simulink model "sensorFusionOfflineHMI"  (R2015b)
settings: Solver=FixedStepDiscrete  StartTime=0.0  StopTime=endTime  FixedStep=0.005  MaxStep=0.005  RelTol=1e-3
values from neighbouring files (symbols this model uses):
  resetStepTime = 500    [main.m]    (also in mainHMI.m)
undefined symbols (not defined in the file or in its folder): EGOSF_CompassHeadingCov, EGOSF_DetectionNorthMax, EGOSF_DetectionNorthMin, EGOSF_GPSHeadingCov, EGOSF_HeadingVelocityLimit, EGOSF_LatAccCov, EGOSF_LatVelInitCov, EGOSF_LonAccCov, EGOSF_LonSpeedCov, EGOSF_OutlierDetection, EGOSF_PhiCov, EGOSF_PhiScale, EGOSF_Pproc, EGOSF_SteeringRatio, EGOSF_YawRateCov, UTMZone
libraries: powerlib_meascontrol x1, sldrtlib x1, etargetslib x1, dspnetwork x1
settings Model: Creator=hultr  LastModifiedBy=axel
settings DataIOCC: SaveFormat=Array
settings DebuggingCC: SolverPrmCheckMsg=warning  InheritedTsInSrcMsg=none  BusObjectLabelMismatch=none
settings HardwareCC: ProdBitPerPointer=32  ProdLargestAtomicFloat=None  ProdIntDivRoundTo=Undefined  ProdEndianess=Unspecified  ProdWordSize=32  ProdHWDeviceType=32-bit Generic
settings GRTTargetCC: GeneratePreprocessorConditionals=Disable all
settings ConfigComp: CovModelRefEnable=Off  CovSFcnEnable=off

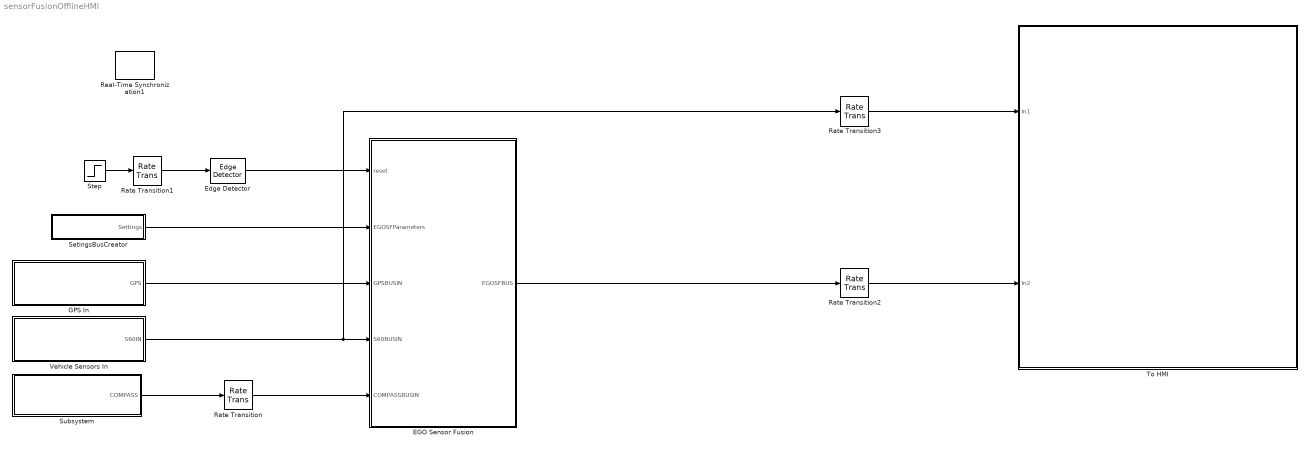
== system sensorFusionOfflineHMI ==
  EGO Sensor Fusion : MATLAB Function  TreatAsAtomicUnit=on  SystemSampleTime=0.025
  Edge Detector : powerlib_meascontrol/Logic/Edge Detector  model=Rising  ic=0  Ts=-1
  GPS In : Subsystem
  Rate Transition : RateTransition
  Rate Transition1 : RateTransition
  Rate Transition2 : RateTransition  OutPortSampleTime=HMIupdateRate
  Rate Transition3 : RateTransition  OutPortSampleTime=HMIupdateRate
  Real-Time Synchronization1 : sldrtlib/Real-Time Synchronization  SampleTime=0.1  MaxMissedTicks=10  ShowMissedTicks=off  YieldWhenWaiting=off
  SetingsBusCreator : Subsystem
  Step : Step  Time=resetStepTime  SampleTime=0
  Subsystem : Subsystem  TreatAsAtomicUnit=on  SystemSampleTime=0.1
  To HMI : Subsystem
  Vehicle Sensors In : Subsystem
  wires:
  Subsystem/1("COMPASS ") -> Rate Transition/1
  GPS In/1(GPS) -> EGO Sensor Fusion/3(GPSBUSIN)
  Vehicle Sensors In/1(S60IN) -> Rate Transition3/1, EGO Sensor Fusion/4(S60BUSIN)
  Step/1 -> Rate Transition1/1
  SetingsBusCreator/1(Settings) -> EGO Sensor Fusion/2(EGOSFParameters)
  Rate Transition/1 -> EGO Sensor Fusion/5(COMPASSBUSIN)
  EGO Sensor Fusion/1(EGOSFBUS) -> Rate Transition2/1
  Edge Detector/1 -> EGO Sensor Fusion/1(reset)
  Rate Transition1/1 -> Edge Detector/1
  Rate Transition3/1 -> To HMI/1(In1)
  Rate Transition2/1 -> To HMI/2(In2)

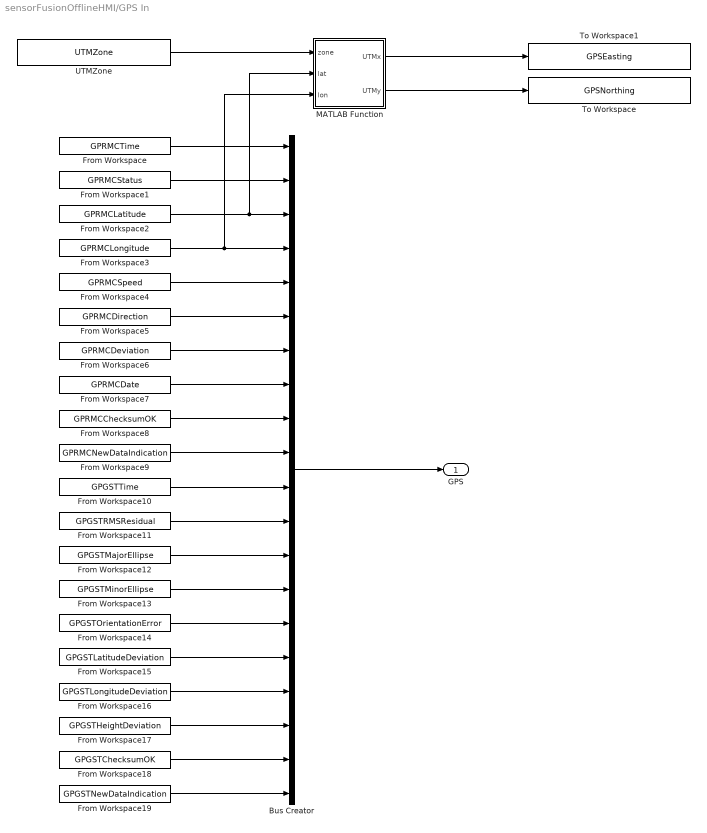
== system sensorFusionOfflineHMI/GPS In ==
  Bus Creator : BusCreator  Inputs=20  OutDataTypeStr=Bus: GPSBUS
  From Workspace : FromWorkspace  VariableName=GPRMCTime  OutDataTypeStr=double  Interpolate=off  OutputAfterFinalValue=Holding final value
  From Workspace1 : FromWorkspace  VariableName=GPRMCStatus  OutDataTypeStr=double  Interpolate=off  OutputAfterFinalValue=Holding final value
  From Workspace10 : FromWorkspace  VariableName=GPGSTTime  OutDataTypeStr=double  Interpolate=off  OutputAfterFinalValue=Holding final value
  From Workspace11 : FromWorkspace  VariableName=GPGSTRMSResidual  OutDataTypeStr=double  Interpolate=off  OutputAfterFinalValue=Holding final value
  From Workspace12 : FromWorkspace  VariableName=GPGSTMajorEllipse  OutDataTypeStr=double  Interpolate=off  OutputAfterFinalValue=Holding final value
  From Workspace13 : FromWorkspace  VariableName=GPGSTMinorEllipse  OutDataTypeStr=double  Interpolate=off  OutputAfterFinalValue=Holding final value
  From Workspace14 : FromWorkspace  VariableName=GPGSTOrientationError  OutDataTypeStr=double  Interpolate=off  OutputAfterFinalValue=Holding final value
  From Workspace15 : FromWorkspace  VariableName=GPGSTLatitudeDeviation  OutDataTypeStr=double  Interpolate=off  OutputAfterFinalValue=Holding final value
  From Workspace16 : FromWorkspace  VariableName=GPGSTLongitudeDeviation  OutDataTypeStr=double  Interpolate=off  OutputAfterFinalValue=Holding final value
  From Workspace17 : FromWorkspace  VariableName=GPGSTHeightDeviation  OutDataTypeStr=double  Interpolate=off  OutputAfterFinalValue=Holding final value
  From Workspace18 : FromWorkspace  VariableName=GPGSTChecksumOK  OutDataTypeStr=double  Interpolate=off  OutputAfterFinalValue=Holding final value
  From Workspace19 : FromWorkspace  VariableName=GPGSTNewDataIndication  OutDataTypeStr=double  Interpolate=off  OutputAfterFinalValue=Holding final value
  From Workspace2 : FromWorkspace  VariableName=GPRMCLatitude  OutDataTypeStr=double  Interpolate=off  OutputAfterFinalValue=Holding final value
  From Workspace3 : FromWorkspace  VariableName=GPRMCLongitude  OutDataTypeStr=double  Interpolate=off  OutputAfterFinalValue=Holding final value
  From Workspace4 : FromWorkspace  VariableName=GPRMCSpeed  OutDataTypeStr=double  Interpolate=off  OutputAfterFinalValue=Holding final value
  From Workspace5 : FromWorkspace  VariableName=GPRMCDirection  OutDataTypeStr=double  Interpolate=off  OutputAfterFinalValue=Holding final value
  From Workspace6 : FromWorkspace  VariableName=GPRMCDeviation  OutDataTypeStr=double  Interpolate=off  OutputAfterFinalValue=Holding final value
  From Workspace7 : FromWorkspace  VariableName=GPRMCDate  OutDataTypeStr=double  Interpolate=off  OutputAfterFinalValue=Holding final value
  From Workspace8 : FromWorkspace  VariableName=GPRMCChecksumOK  OutDataTypeStr=double  Interpolate=off  OutputAfterFinalValue=Holding final value
  From Workspace9 : FromWorkspace  VariableName=GPRMCNewDataIndication  OutDataTypeStr=double  Interpolate=off  OutputAfterFinalValue=Holding final value
  MATLAB Function : MATLAB Function  TreatAsAtomicUnit=on
  To Workspace : ToWorkspace  VariableName=GPSNorthing  SaveFormat=Structure With Time  SampleTime=-1
  To Workspace1 : ToWorkspace  VariableName=GPSEasting  SaveFormat=Structure With Time  SampleTime=-1
  UTMZone : Constant  Value=UTMZone  SampleTime=-1
  GPS : Outport
  wires:
  From Workspace/1 -> Bus Creator/1
  Bus Creator/1 -> GPS/1
  From Workspace1/1 -> Bus Creator/2
  From Workspace2/1 -> MATLAB Function/2(lat), Bus Creator/3
  From Workspace3/1 -> MATLAB Function/3(lon), Bus Creator/4
  From Workspace4/1 -> Bus Creator/5
  From Workspace5/1 -> Bus Creator/6
  From Workspace6/1 -> Bus Creator/7
  From Workspace7/1 -> Bus Creator/8
  From Workspace8/1 -> Bus Creator/9
  From Workspace9/1 -> Bus Creator/10
  From Workspace10/1 -> Bus Creator/11
  From Workspace11/1 -> Bus Creator/12
  From Workspace12/1 -> Bus Creator/13
  From Workspace13/1 -> Bus Creator/14
  From Workspace14/1 -> Bus Creator/15
  From Workspace15/1 -> Bus Creator/16
  From Workspace16/1 -> Bus Creator/17
  From Workspace17/1 -> Bus Creator/18
  From Workspace18/1 -> Bus Creator/19
  From Workspace19/1 -> Bus Creator/20
  MATLAB Function/2(UTMy) -> To Workspace/1
  MATLAB Function/1(UTMx) -> To Workspace1/1
  UTMZone/1 -> MATLAB Function/1(zone)

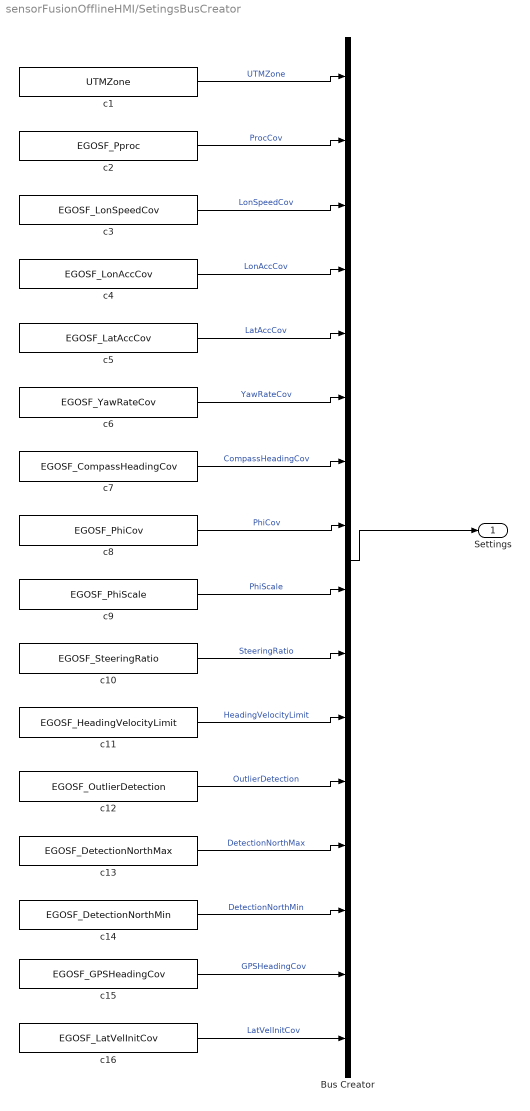
== system sensorFusionOfflineHMI/SetingsBusCreator ==
  Bus Creator : BusCreator  Inputs=16  OutDataTypeStr=Bus: EGOSFSETTINGS
  c1 : Constant  Value=UTMZone  SampleTime=-1
  c10 : Constant  Value=EGOSF_SteeringRatio  SampleTime=-1
  c11 : Constant  Value=EGOSF_HeadingVelocityLimit  SampleTime=-1
  c12 : Constant  Value=EGOSF_OutlierDetection  SampleTime=-1
  c13 : Constant  Value=EGOSF_DetectionNorthMax  SampleTime=-1
  c14 : Constant  Value=EGOSF_DetectionNorthMin  SampleTime=-1
  c15 : Constant  Value=EGOSF_GPSHeadingCov  SampleTime=-1
  c16 : Constant  Value=EGOSF_LatVelInitCov  SampleTime=-1
  c2 : Constant  Value=EGOSF_Pproc  SampleTime=-1
  c3 : Constant  Value=EGOSF_LonSpeedCov  SampleTime=-1
  c4 : Constant  Value=EGOSF_LonAccCov  SampleTime=-1
  c5 : Constant  Value=EGOSF_LatAccCov  SampleTime=-1
  c6 : Constant  Value=EGOSF_YawRateCov  SampleTime=-1
  c7 : Constant  Value=EGOSF_CompassHeadingCov  SampleTime=-1
  c8 : Constant  Value=EGOSF_PhiCov  SampleTime=-1
  c9 : Constant  Value=EGOSF_PhiScale  SampleTime=-1
  Settings : Outport
  wires:
  Bus Creator/1 -> Settings/1
  c1/1 -> Bus Creator/1  "UTMZone"
  c2/1 -> Bus Creator/2  "ProcCov"
  c3/1 -> Bus Creator/3  "LonSpeedCov"
  c4/1 -> Bus Creator/4  "LonAccCov"
  c6/1 -> Bus Creator/6  "YawRateCov"
  c7/1 -> Bus Creator/7  "CompassHeadingCov"
  c5/1 -> Bus Creator/5  "LatAccCov"
  c8/1 -> Bus Creator/8  "PhiCov"
  c9/1 -> Bus Creator/9  "PhiScale"
  c10/1 -> Bus Creator/10  "SteeringRatio"
  c11/1 -> Bus Creator/11  "HeadingVelocityLimit"
  c12/1 -> Bus Creator/12  "OutlierDetection"
  c13/1 -> Bus Creator/13  "DetectionNorthMax"
  c14/1 -> Bus Creator/14  "DetectionNorthMin"
  c15/1 -> Bus Creator/15  "GPSHeadingCov"
  c16/1 -> Bus Creator/16  "LatVelInitCov"

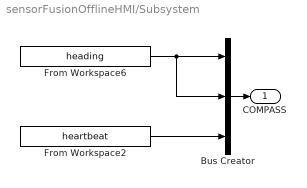
== system sensorFusionOfflineHMI/Subsystem ==
  Bus Creator : BusCreator  Inputs=3  OutDataTypeStr=Bus: COMPASSBUS
  From Workspace2 : FromWorkspace  VariableName=heartbeat  OutDataTypeStr=double
  From Workspace6 : FromWorkspace  VariableName=heading  OutDataTypeStr=double
  "COMPASS " : Outport
  wires:
  From Workspace2/1 -> Bus Creator/3
  From Workspace6/1 -> Bus Creator/2, Bus Creator/1
  Bus Creator/1 -> "COMPASS "/1

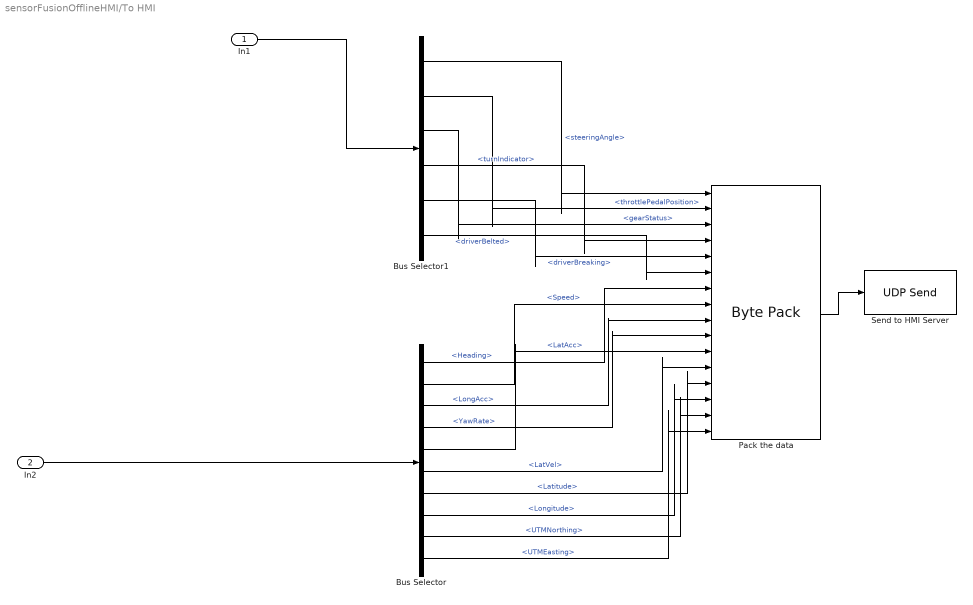
== system sensorFusionOfflineHMI/To HMI ==
  In1 : Inport
  In2 : Inport  Port=2
  Bus Selector : BusSelector  OutputSignals=Heading,Speed,LongAcc,YawRate,LatAcc,LatVel,Latitude,Longitude,UTMNorthing,UTMEasting
  Bus Selector1 : BusSelector  OutputSignals=steeringAngle,throttlePedalPosition,gearStatus,turnIndicator,driverBreaking,driverBelted
  Pack the data : etargetslib/Byte Pack  datatypes={'double', 'double', 'double', 'double', 'double', 'double', 'double', 'double', 'double', 'double', 'double', 'double', 'double', 'double', 'double', 'double'}  byteAlign=1
  Send to HMI Server : dspnetwork/UDP Send  remoteURL='0.0.0.0'  remotePort=41234  localURL='0.0.0.0'  localPortSource=Automatically determine  localPort=-1  sampletime=-1  separateLengthPort=0
  wires:
  Bus Selector1/6 -> Pack the data/6  "<driverBelted>"
  Bus Selector/6 -> Pack the data/12  "<LatVel>"
  Bus Selector1/5 -> Pack the data/5  "<driverBreaking>"
  In2/1 -> Bus Selector/1
  Bus Selector1/2 -> Pack the data/2  "<throttlePedalPosition>"
  In1/1 -> Bus Selector1/1
  Bus Selector/1 -> Pack the data/7  "<Heading>"
  Bus Selector/2 -> Pack the data/8  "<Speed>"
  Bus Selector1/3 -> Pack the data/3  "<gearStatus>"
  Bus Selector1/4 -> Pack the data/4  "<turnIndicator>"
  Bus Selector/5 -> Pack the data/11  "<LatAcc>"
  Bus Selector/4 -> Pack the data/10  "<YawRate>"
  Bus Selector1/1 -> Pack the data/1  "<steeringAngle>"
  Bus Selector/3 -> Pack the data/9  "<LongAcc>"
  Pack the data/1 -> Send to HMI Server/1
  Bus Selector/7 -> Pack the data/13  "<Latitude>"
  Bus Selector/8 -> Pack the data/14  "<Longitude>"
  Bus Selector/9 -> Pack the data/15  "<UTMNorthing>"
  Bus Selector/10 -> Pack the data/16  "<UTMEasting>"

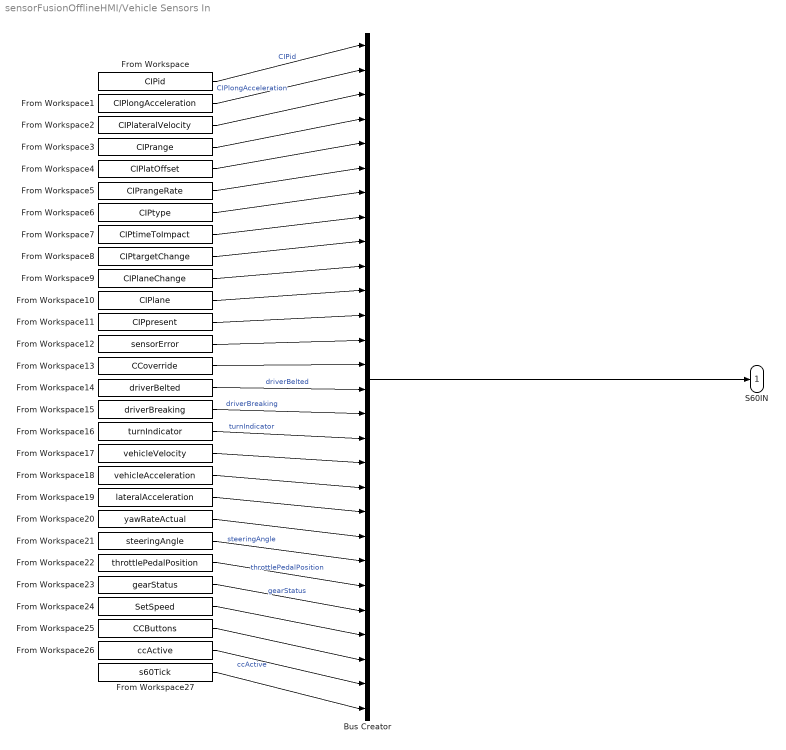
== system sensorFusionOfflineHMI/Vehicle Sensors In ==
  Bus Creator : BusCreator  Inputs=28  OutDataTypeStr=Bus: S60OUTBUS  NonVirtualBus=on
  From Workspace : FromWorkspace  VariableName=CIPid  OutDataTypeStr=double  SampleTime=0.025
  From Workspace1 : FromWorkspace  VariableName=CIPlongAcceleration  SampleTime=0.025
  From Workspace10 : FromWorkspace  VariableName=CIPlane  SampleTime=0.025
  From Workspace11 : FromWorkspace  VariableName=CIPpresent  SampleTime=0.025
  From Workspace12 : FromWorkspace  VariableName=sensorError  SampleTime=0.025
  From Workspace13 : FromWorkspace  VariableName=CCoverride  SampleTime=0.025
  From Workspace14 : FromWorkspace  VariableName=driverBelted  SampleTime=0.025
  From Workspace15 : FromWorkspace  VariableName=driverBreaking  SampleTime=0.025
  From Workspace16 : FromWorkspace  VariableName=turnIndicator  SampleTime=0.025
  From Workspace17 : FromWorkspace  VariableName=vehicleVelocity  SampleTime=0.025
  From Workspace18 : FromWorkspace  VariableName=vehicleAcceleration  SampleTime=0.025
  From Workspace19 : FromWorkspace  VariableName=lateralAcceleration  SampleTime=0.025
  From Workspace2 : FromWorkspace  VariableName=CIPlateralVelocity  SampleTime=0.025
  From Workspace20 : FromWorkspace  VariableName=yawRateActual  SampleTime=0.025
  From Workspace21 : FromWorkspace  VariableName=steeringAngle  SampleTime=0.025
  From Workspace22 : FromWorkspace  VariableName=throttlePedalPosition  SampleTime=0.025
  From Workspace23 : FromWorkspace  VariableName=gearStatus  SampleTime=0.025
  From Workspace24 : FromWorkspace  VariableName=SetSpeed  SampleTime=0.025
  From Workspace25 : FromWorkspace  VariableName=CCButtons  SampleTime=0.025
  From Workspace26 : FromWorkspace  VariableName=ccActive  SampleTime=0.025
  From Workspace27 : FromWorkspace  VariableName=s60Tick  SampleTime=0.025
  From Workspace3 : FromWorkspace  VariableName=CIPrange  SampleTime=0.025
  From Workspace4 : FromWorkspace  VariableName=CIPlatOffset  SampleTime=0.025
  From Workspace5 : FromWorkspace  VariableName=CIPrangeRate  SampleTime=0.025
  From Workspace6 : FromWorkspace  VariableName=CIPtype  SampleTime=0.025
  From Workspace7 : FromWorkspace  VariableName=CIPtimeToImpact  SampleTime=0.025
  From Workspace8 : FromWorkspace  VariableName=CIPtargetChange  SampleTime=0.025
  From Workspace9 : FromWorkspace  VariableName=CIPlaneChange  SampleTime=0.025
  S60IN : Outport
  wires:
  Bus Creator/1 -> S60IN/1
  From Workspace/1 -> Bus Creator/1  "CIPid"
  From Workspace1/1 -> Bus Creator/2  "CIPlongAcceleration"
  From Workspace2/1 -> Bus Creator/3
  From Workspace3/1 -> Bus Creator/4
  From Workspace4/1 -> Bus Creator/5
  From Workspace5/1 -> Bus Creator/6
  From Workspace6/1 -> Bus Creator/7
  From Workspace7/1 -> Bus Creator/8
  From Workspace8/1 -> Bus Creator/9
  From Workspace9/1 -> Bus Creator/10
  From Workspace10/1 -> Bus Creator/11
  From Workspace11/1 -> Bus Creator/12
  From Workspace13/1 -> Bus Creator/14
  From Workspace12/1 -> Bus Creator/13
  From Workspace23/1 -> Bus Creator/24  "gearStatus"
  From Workspace17/1 -> Bus Creator/18
  From Workspace18/1 -> Bus Creator/19
  From Workspace20/1 -> Bus Creator/21
  From Workspace21/1 -> Bus Creator/22  "steeringAngle"
  From Workspace16/1 -> Bus Creator/17  "turnIndicator"
  From Workspace15/1 -> Bus Creator/16  "driverBreaking"
  From Workspace25/1 -> Bus Creator/26
  From Workspace19/1 -> Bus Creator/20
  From Workspace24/1 -> Bus Creator/25
  From Workspace14/1 -> Bus Creator/15  "driverBelted"
  From Workspace22/1 -> Bus Creator/23  "throttlePedalPosition"
  From Workspace26/1 -> Bus Creator/27  "ccActive"
  From Workspace27/1 -> Bus Creator/28

== matlab function sensorFusionOfflineHMI/EGO Sensor Fusion ==
  data: reset input; EGOSFParameters input Bus: EGOSFSETTINGS; GPSBUSIN input Bus: GPSBUS; EGOSFBUS output Bus: EGOSFBUS; S60BUSIN input Bus: S60OUTBUS; COMPASSBUSIN input Bus: COMPASSBUS
function EGOSFBUS = fcn(reset,EGOSFParameters,GPSBUSIN,S60BUSIN,COMPASSBUSIN)
%#codegen
% =========================================================================
% GCDC Sensor fusion offline template. Modify as needed
% Robert Hult, 10/3-16
%
% SOME RECOMMENDATIONS:
%  - in the update steps, build the measurment equations "on the fly"
%    depending on which sensors has new data
%  - Include a validity-check on the GPS data, outliers are relatively
%    common, especially when using the correction
%  - Take care with angles! be aware that things might get weird du to mod
%    2Pi. This MUST be handled in some waym otherwsie we will get weird
%    behaviour.
%  - NOTE: All measurments are NOT given in SI units
%
% =========================================================================
% Dummy example implementation using unicycle kinematics
% State X = [x,y,vlon,alon,vlat,alat,yaw,yawrate,phi]
nStates = 9;
persistent X 
if isempty(X)
    X = zeros(nStates,1);
end

persistent P
if isempty(P)
    P = zeros(nStates);
end

%%%%%%%%%%%%%%%%%%%%%%%%%%%%%%%%%%%%%%%%%%%%%%%%%%%%%%%%%%%%%%%%%%%%%%%%%%%
%%%%%%%%%%%%%%%%%%%% DATA CHECKING %%%%%%%%%%%%%%%%%%%%%%%%%%%%%%%%%%%%%%%%
%%%%%%%%%%%%%%%%%%%%%%%%%%%%%%%%%%%%%%%%%%%%%%%%%%%%%%%%%%%%%%%%%%%%%%%%%%%
% CHECK GPS DATA
persistent timeAtPreviousGPSreading
if isempty(timeAtPreviousGPSreading)
    timeAtPreviousGPSreading = 0;
end

if GPSBUSIN.GPRMCTime == timeAtPreviousGPSreading || GPSBUSIN.GPRMCStatus ~= 1
   UTMx             = NaN;
   UTMy             = NaN;
   GpsCov           = NaN(2);
   newGPSData       = 0;
else
% FUNCTIONS FOUND IN AUXILARY FOLDER
% Decimal degrees to DEG,Min,sec.decsec
[Latdec,Londec]= dm2deg(GPSBUSIN.GPRMCLatitude,GPSBUSIN.GPRMCLongitude);
% Decimal degrees to UTM approximation
[UTMx, UTMy] = wgs2utm(Latdec,Londec,EGOSFParameters.UTMZone);
% Convert Covariance
GpsCov=gpscov(GPSBUSIN.GPGSTMajorEllipse,GPSBUSIN.GPGSTMinorEllipse,GPSBUSIN.GPGSTOrientationError);
newGPSData = 1;
end


% =========================================================================
% =========================================================================
% CHECK S60 DATA
persistent tickAtPreviousS60Reading
if isempty(tickAtPreviousS60Reading)
    tickAtPreviousS60Reading = 0;
end

if tickAtPreviousS60Reading ~= S60BUSIN.s60Tick
    tickAtPreviousS60Reading = S60BUSIN.s60Tick;
    newS60Data = 1;
else
    newS60Data = 0;
end

% =========================================================================
% =========================================================================
% CHECK COMPASS DATA
persistent tickAtPreviousCompassReading
if isempty(tickAtPreviousCompassReading)
    tickAtPreviousCompassReading = 0;
end

if tickAtPreviousCompassReading ~= COMPASSBUSIN.heartbeat
    tickAtPreviousCompassReading = COMPASSBUSIN.heartbeat;
    newCompassData = 1;
else
    newCompassData = 0;
end

%%%%%%%%%%%%%%%%%%%%%%%%%%%%%%%%%%%%%%%%%%%%%%%%%%%%%%%%%%%%%%%%%%%%%%%%%%%
%%%%%%%%%%%%%%%% FILTER MANAGEMENT LOGIC  %%%%%%%%%%%%%%%%%%%%%%%%%%%%%%%%%
%%%%%%%%%%%%%%%%%%%%%%%%%%%%%%%%%%%%%%%%%%%%%%%%%%%%%%%%%%%%%%%%%%%%%%%%%%%
% 1) Enables resetting of state and covariances
% 2) Initializes the states as the sensor values on reset.
% 3) Initializes the position when new GPS data comes in, otherwise freezes
%    it on the last recieved position (completely arbitrary)
% -------------------------------------------------------------------------
persistent positionIsInitialized
if isempty(positionIsInitialized) 
   positionIsInitialized = 0; 
end

persistent statesAreInitialized
if isempty(statesAreInitialized) 
    statesAreInitialized = 0;
end

if reset == 1
    positionIsInitialized = 0;
    statesAreInitialized = 0;
end




if statesAreInitialized == 0
   % Reset State, reset covariance
   X = X*0;
   P = P*0;
   P(1,1) = 1e6;
   P(2,2) = 1e6;
   P(2,1) = 1e6;
   P(1,2) = 1e6;
   P(3,3) = EGOSFParameters.LonSpeedCov;
   P(4,4) = EGOSFParameters.LonAccCov;
   P(5,5) = EGOSFParameters.LatVelInitCov;
   P(6,6) = EGOSFParameters.LatAccCov;
   P(7,7) = EGOSFParameters.CompassHeadingCov;
   P(8,8) = EGOSFParameters.YawRateCov;
   P(9,9) = EGOSFParameters.PhiCov;
 
   X(3) = S60BUSIN.vehicleVelocity;
   X(4) = S60BUSIN.vehicleAcceleration;
   X(5) = COMPASSBUSIN.heading*pi/180;
   X(6) = S60BUSIN.lateralAcceleration;
   X(7) = GPSBUSIN.GPRMCDirection;
   X(8) = S60BUSIN.yawRateActual;
   X(9) = (S60BUSIN.steeringAngle*pi/180)/EGOSFParameters.SteeringRatio;
   
   statesAreInitialized = 1;
end

if positionIsInitialized == 0
    if newGPSData
        if S60BUSIN.vehicleVelocity > EGOSFParameters.HeadingVelocityLimit 
            X(5)   =  (2*pi -GPSBUSIN.GPRMCDirection*pi/180);
            P(5,5) = EGOSFParameters.GPSHeadingCov;
        end
        X(1) = UTMx;
        X(2) = UTMy;
        P(1:2,1:2) = GpsCov;
        positionIsInitialized = 1;    
    end
end

%%%%%%%%%%%%%%%%%%%%%%%%%%%%%%%%%%%%%%%%%%%%%%%%%%%%%%%%%%%%%%%%%%%%%%%%%%%
%%%%%%%%%%%%%%%%%%%%% PREDICTION-CORRECTION %%%%%%%%%%%%%%%%%%%%%%%%%%%%%%%
%%%%%%%%%%%%%%%%%%%%%%%%%%%%%%%%%%%%%%%%%%%%%%%%%%%%%%%%%%%%%%%%%%%%%%%%%%%

% PREDICTION
if abs(X(3))<0.01
    X(3)=0.01;
end

X  = dynamicsFun(X);
dF = jacobianFun(X); 
P  =  dF*P*dF' + EGOSFParameters.ProcCov;

% CORRECTION (Assumption is that vehicle allways give new data)
yMeasured  = [UTMx; UTMy; S60BUSIN.vehicleVelocity; S60BUSIN.vehicleAcceleration; S60BUSIN.lateralAcceleration; (2*pi -GPSBUSIN.GPRMCDirection*pi/180); S60BUSIN.yawRateActual*pi/180; +(S60BUSIN.steeringAngle*pi/180)/EGOSFParameters.SteeringRatio  ]; % -(COMPASSBUSIN.heading)+2*pi  GPSBUSIN.GPRMCDirection*pi/180 -(2*pi -GPSBUSIN.GPRMCDirection*pi/180)
tmp = eye(9);
I = [(1:4),(6:9)];
H = tmp(I,:);
H(8,9) = EGOSFParameters.PhiScale;

yEstimate  = H*X; 

Rconst = diag([EGOSFParameters.LonSpeedCov,...
               EGOSFParameters.LonAccCov,...
               EGOSFParameters.LatAccCov,...
               EGOSFParameters.GPSHeadingCov,...
               EGOSFParameters.YawRateCov,...            %EGOSFParameters.CompassHeadingCov 0.1*GPSBUSIN.GPGSTOrientationError*pi/180
               EGOSFParameters.PhiCov]);
           
R = blkdiag(GpsCov,Rconst);

X_e = [ yEstimate(1)-yMeasured(1); yEstimate(2)-yMeasured(2)];                              %Error of position

if newGPSData
    
    if S60BUSIN.vehicleVelocity >= EGOSFParameters.HeadingVelocityLimit 
        I = 1:8;
    else
        I = [1,2,3,4,5,7,8];
    end
    
    if sqrt(X_e'*X_e)>EGOSFParameters.OutlierDetection  %X_e'/(P(1:2,1:2))*X_e>2
        I=I(3:end);
    end
    
else
    I = [3,4,5,6,8];
end

up = 0;
if newGPSData && X(7)>EGOSFParameters.DetectionNorthMax && yMeasured(6)<EGOSFParameters.DetectionNorthMin
    yMeasured(6) = 2*pi + yMeasured(6);
    up=1;
elseif newGPSData && X(7)<EGOSFParameters.DetectionNorthMin && yMeasured(6)>EGOSFParameters.DetectionNorthMax
    yMeasured(6) = -2*pi + yMeasured(6);
    up=1;
end

innovation = yMeasured(I)-yEstimate(I); 

S = H(I,:)*P*(H(I,:))' + R(I,I);

K = P*(H(I,:)'/S);
X = X + K*innovation;
P = (eye(nStates) - K*H(I,:))*P;

X(7) = mod(X(7),2*pi);


%%%%%%%%%%%%%%%%%%%%%%%%%%%%%%%%%%%%%%%%%%%%%%%%%%%%%%%%%%%%%%%%%%%%%%%%%%%
%%%%%%%%%%%%%%%%%%%%% OUTPUT FORMATTING %%%%%%%%%%%%%%%%%%%%%%%%%%%%%%%%%%%
%%%%%%%%%%%%%%%%%%%%%%%%%%%%%%%%%%%%%%%%%%%%%%%%%%%%%%%%%%%%%%%%%%%%%%%%%%%
% NOTE THAT SIGNALS MUCH BE DEFINED IN THE ORDER IT APPEARS IN THE BUS

[Lat,Lon]=utm2wgs(X(1),X(2),EGOSFParameters.UTMZone);
[SemiMajor,SemiMinor,Theta]= ErrorEllipse2(P(1:2,1:2));

EGOSFBUS.UTMNorthing            = X(2);
EGOSFBUS.UTMEasting             = X(1);
EGOSFBUS.Latitude               = Lat; 
EGOSFBUS.Longitude              = Lon; 
EGOSFBUS.SemiMajorConfidence 	= SemiMajor; 
EGOSFBUS.SemiMinorConfidence    = SemiMinor; 
EGOSFBUS.SemiMajorOrientation   = Theta; 
EGOSFBUS.Altitude               = 0;        % Needed?
EGOSFBUS.Heading                = X(7);
EGOSFBUS.HeadingConfidence      = 2*sqrt(P(7,7));
EGOSFBUS.Speed                  = X(3);
EGOSFBUS.SpeedConfidence        = 2*sqrt(P(3,3));
EGOSFBUS.LongAcc                = X(4);
EGOSFBUS.LongAccConfidence      = 2*sqrt(P(4,4));
EGOSFBUS.YawRate                = X(8);
EGOSFBUS.YawRateConfidence      = 2*sqrt(P(8,8));
EGOSFBUS.LatAcc                 = X(6); 
EGOSFBUS.LatVel                 = X(5); 
end

== matlab function sensorFusionOfflineHMI/GPS In/MATLAB Function ==
  data: zone input; UTMx output; lat input; UTMy output; lon input
function [UTMx,UTMy] = fcn(zone,lat,lon)
%#codegen


[Latdec,Londec]= dm2deg(lat,lon);
% Decimal degrees to UTM approximation
[UTMx, UTMy] = wgs2utm(Latdec,Londec,zone);
